simulink model "control_motor"  (R2017b)
settings: Solver=VariableStepAuto  StartTime=0.0  StopTime=0.15  RelTol=1e-3
settings Model: Creator=jinpa  LastModifiedBy=jinpa

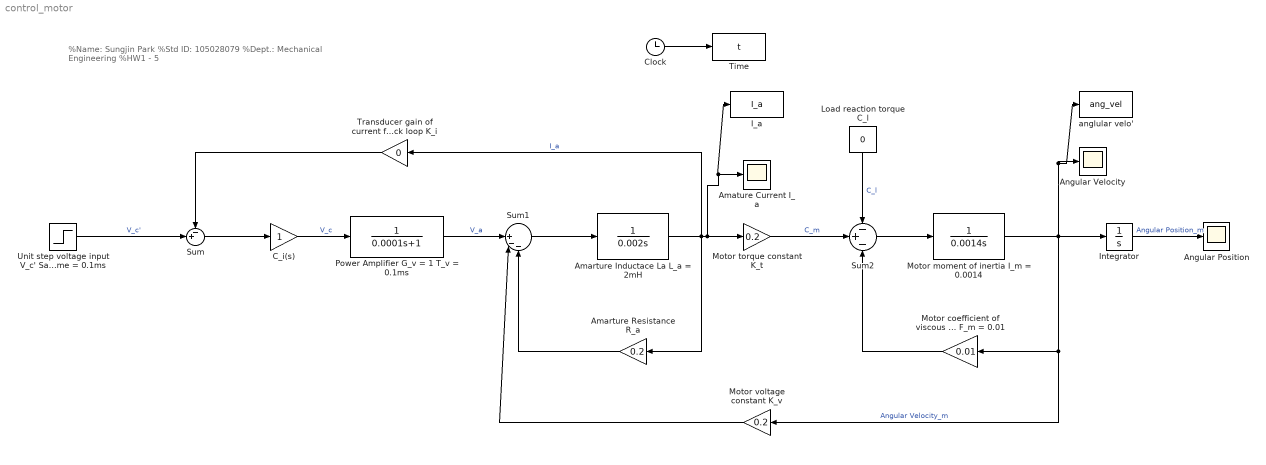
== system control_motor ==
  note: %Name: Sungjin Park
      | %Std ID: 105028079
      | %Dept.: Mechanical Engineering
      |
      | %HW1 - 5
  " I_a" : ToWorkspace  VariableName=I_a  SaveFormat=Timeseries  SampleTime=0.0001
  Amarture Inductace La L_a = 2mH : TransferFcn  Denominator=[0.002 0]
  Amarture Resistance R_a : Gain  Gain=0.2
  Amature Current I_a : Scope
  Angular Position : Scope
  Angular Velocity : Scope
  C_i(s) : Gain
  Clock : Clock
  Integrator : Integrator
  Load reaction torque C_l : Constant  Value=0  SampleTime=0.0001
  Motor coefficient of viscous friction F_m = 0.01 : Gain  Gain=0.01
  Motor moment of inertia I_m = 0.0014 : TransferFcn  Denominator=[0.0014 0]
  Motor torque constant K_t : Gain  Gain=0.2
  Motor voltage constant K_v : Gain  Gain=0.2
  Power Amplifier G_v = 1 T_v = 0.1ms : TransferFcn  Denominator=[0.0001 1]
  Sum : Sum  Inputs=-+|
  Sum1 : Sum  Inputs=||+--
  Sum2 : Sum  Inputs=-+-
  Time : ToWorkspace  VariableName=t  SaveFormat=Timeseries  SampleTime=0.0001
  Transducer gain of current feedback loop K_i : Gain  Gain=0
  Unit step voltage input V_c' Sampling time = 0.1ms : Step  Before=1  SampleTime=0.0001
  anglular velo' : ToWorkspace  VariableName=ang_vel  SaveFormat=Timeseries  SampleTime=0.0001
  wires:
  Unit step voltage input V_c' Sampling time = 0.1ms/1 -> Sum/2  "V_c'"
  Integrator/1 -> Angular Position/1  "Angular Position_m"
  Motor moment of inertia I_m = 0.0014/1 -> Motor coefficient of viscous friction F_m = 0.01/1, Motor voltage constant K_v/1, Integrator/1, anglular velo'/1, Angular Velocity/1  "Angular Velocity_m"
  Sum/1 -> C_i(s)/1
  C_i(s)/1 -> Power Amplifier G_v = 1 T_v = 0.1ms/1  "V_c"
  Power Amplifier G_v = 1 T_v = 0.1ms/1 -> Sum1/1  "V_a"
  Sum1/1 -> Amarture Inductace La L_a = 2mH/1
  Amarture Inductace La L_a = 2mH/1 -> Amarture Resistance R_a/1, Transducer gain of current feedback loop K_i/1, Motor torque constant K_t/1, " I_a"/1, Amature Current I_a/1  "I_a"
  Motor torque constant K_t/1 -> Sum2/2  "C_m"
  Sum2/1 -> Motor moment of inertia I_m = 0.0014/1
  Transducer gain of current feedback loop K_i/1 -> Sum/1
  Amarture Resistance R_a/1 -> Sum1/3
  Motor voltage constant K_v/1 -> Sum1/2
  Motor coefficient of viscous friction F_m = 0.01/1 -> Sum2/3
  Load reaction torque C_l/1 -> Sum2/1  "C_l"
  Clock/1 -> Time/1
